simulink library "PI_library"  (R2020b)
settings: Solver=VariableStepAuto  StartTime=0.0  StopTime=10.0  RelTol=1e-3
settings Model: Creator=vijay jagtap  LastModifiedBy=vijay jagtap

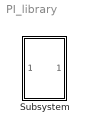
== system PI_library ==
  Subsystem : Subsystem  mask{Kp=25, Ki=300, Ts=0.01}
      mask Display: image('download.jpg'); % Use "Edit Image" on toolstrip to change.

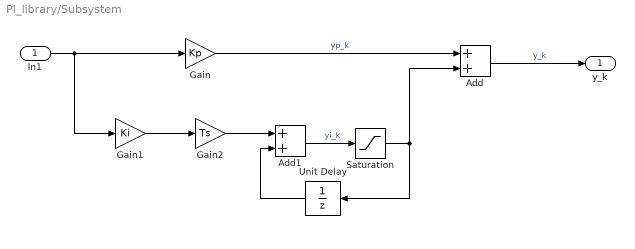
== system PI_library/Subsystem ==
  In1 : Inport
  Add : Sum
  Add1 : Sum
  Gain : Gain  Gain=Kp
  Gain1 : Gain  Gain=Ki
  Gain2 : Gain  Gain=Ts
  Saturation : Saturate  UpperLimit=1  LowerLimit=-1
  Unit Delay : UnitDelay  SampleTime=-1  HasFrameUpgradeWarning=on
  y_k : Outport
  wires:
  In1/1 -> Gain/1, Gain1/1
  Unit Delay/1 -> Add1/2
  Add1/1 -> Saturation/1  "yi_k"
  Add/1 -> y_k/1  "y_k"
  Gain2/1 -> Add1/1
  Gain/1 -> Add/1  "yp_k"
  Gain1/1 -> Gain2/1
  Saturation/1 -> Unit Delay/1, Add/2
